simulink model "PowertaskEM22_Quadra"  (R2023b)
settings: Solver=VariableStepAuto  StartTime=0.0  StopTime=1  RelTol=1e-3
libraries: spsThreePhaseTransformerTwoWindingsLib x5, spsThreePhaseParallelRLCBranchLib x4, spsThreePhaseBreakerLib x4, spsThreePhaseVIMeasurementLib x4, spsRMSLib x4, spsThreePhaseSourceLib x3, sps_lib x1
settings Model: Creator=Shanilka T. Yapa  LastModifiedBy=Shanilka T. Yapa

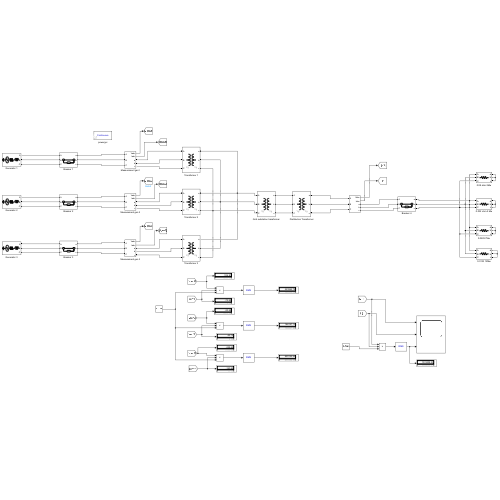
[thumbnail: Simulink's stored preview of the top-level diagram]
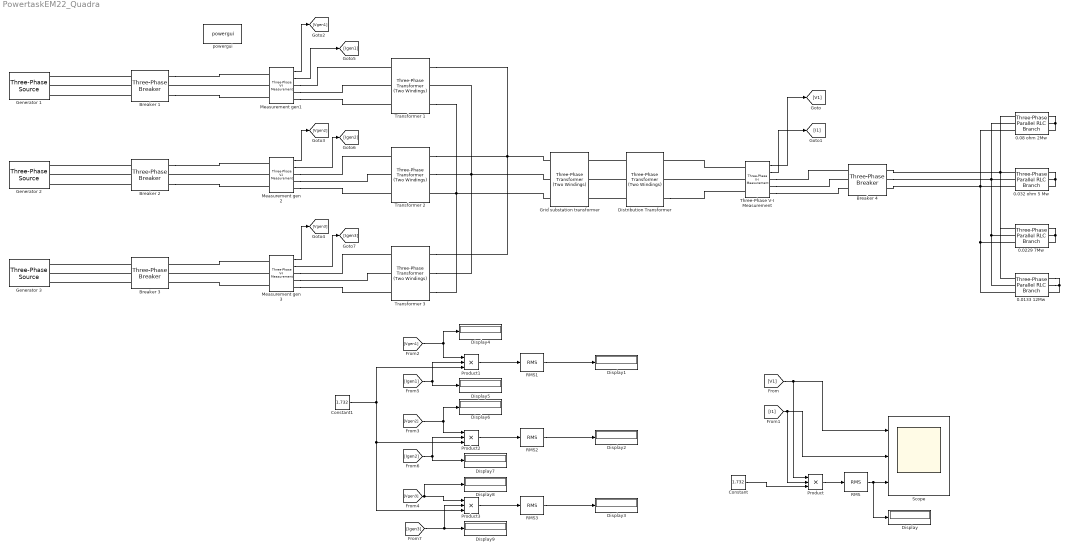
== system PowertaskEM22_Quadra ==
  0.0133 12Mw : spsThreePhaseParallelRLCBranchLib/Three-Phase Parallel RLC Branch  LConnTagsString=A|B|C  RConnTagsString=A|B|C  BranchType=R  Resistance=0.0133  Inductance=1e-3  Capacitance=1e-6  Measurements=None
  0.0229 7Mw : spsThreePhaseParallelRLCBranchLib/Three-Phase Parallel RLC Branch  LConnTagsString=A|B|C  RConnTagsString=A|B|C  BranchType=R  Resistance=0.0229  Inductance=1e-3  Capacitance=1e-6  Measurements=None
  0.032 ohm 5 Mw : spsThreePhaseParallelRLCBranchLib/Three-Phase Parallel RLC Branch  LConnTagsString=A|B|C  RConnTagsString=A|B|C  BranchType=R  Resistance=0.032  Inductance=0  Capacitance=0  Measurements=None
  0.08 ohm 2Mw : spsThreePhaseParallelRLCBranchLib/Three-Phase Parallel RLC Branch  LConnTagsString=A|B|C  RConnTagsString=A|B|C  BranchType=R  Resistance=0.08  Inductance=0  Capacitance=0  Measurements=None
  Breaker {1..4} (4 alike) : spsThreePhaseBreakerLib/Three-Phase Breaker  InitialState=closed  SwitchA=on  SwitchB=on  SwitchC=on  SwitchTimes="[1/60  5/60]"  External=off  BreakerResistance=0.01  SnubberResistance=1e6  SnubberCapacitance=inf  Measurements=None
  Constant : Constant  Value=1.732
  Constant1 : Constant  Value=1.732
  Display{,1..9} (10 alike) : Display
      settings: Format=bank
  Distribution Transformer : spsThreePhaseTransformerTwoWindingsLib/Three-Phase Transformer (Two Windings)  Winding1Connection=Yg  Winding2Connection=Yg  CoreType=Three single-phase transformers  SetSaturation=off  Hysteresis=off  DataFile='hysteresis'  SetInitialFlux=off  Measurements=None  UNITS=SI  NominalPower=[ 3e6 , 50 ]  Winding1=[11e3, 0.2, 0.006]  Winding2=[400, 0.001, 1e-4]  Rm=1e5  Lm=1e5  L0=0.5  Saturation=[0 0;0.66653 1910.3;277.72 2419.7]  InitialFluxes=[ 0.8 , -0.8 , 0.7 ]  BreakLoop=off  DiscreteSolver=Trapezoidal iterative  DataType=on  TransfoNumber=1
  Generator 1 : spsThreePhaseSourceLib/Three-Phase Source  InternalConnection=Yg  VoltagePhases=off  Voltage=11e3  PhaseAngle=0  Voltage_phases=[25e3 25e3 25e3]/sqrt(3)  PhaseAngles_phases=[0 -120 +120]  Frequency=50  NonIdealSource=on  SpecifyImpedance=off  Resistance=0.8929  Inductance=16.58e-3  ShortCircuitLevel=100e6  BaseVoltage=25e3  XRratio=7  BusType=PV  Pref=1e6  Qref=0  Prefabc=[10e3, 10e3, 10e3]  Qrefabc=[0, 0, 0]  Qmin=-inf  Qmax=inf
  Generator 2 : spsThreePhaseSourceLib/Three-Phase Source  InternalConnection=Yg  VoltagePhases=off  Voltage=12e3  PhaseAngle=0  Voltage_phases=[25e3 25e3 25e3]/sqrt(3)  PhaseAngles_phases=[0 -120 +120]  Frequency=50  NonIdealSource=on  SpecifyImpedance=off  Resistance=0.8929  Inductance=16.58e-3  ShortCircuitLevel=100e6  BaseVoltage=25e3  XRratio=7  BusType=PV  Pref=2e6  Qref=0  Prefabc=[10e3, 10e3, 10e3]  Qrefabc=[0, 0, 0]  Qmin=-inf  Qmax=inf
  Generator 3 : spsThreePhaseSourceLib/Three-Phase Source  InternalConnection=Yg  VoltagePhases=off  Voltage=10e3  PhaseAngle=0  Voltage_phases=[25e3 25e3 25e3]/sqrt(3)  PhaseAngles_phases=[0 -120 +120]  Frequency=50  NonIdealSource=on  SpecifyImpedance=off  Resistance=0.8929  Inductance=16.58e-3  ShortCircuitLevel=100e6  BaseVoltage=25e3  XRratio=7  BusType=PV  Pref=4e6  Qref=0  Prefabc=[10e3, 10e3, 10e3]  Qrefabc=[0, 0, 0]  Qmin=-inf  Qmax=inf
  Grid substation transformer : spsThreePhaseTransformerTwoWindingsLib/Three-Phase Transformer (Two Windings)  Winding1Connection=Yg  Winding2Connection=Yg  CoreType=Three single-phase transformers  SetSaturation=off  Hysteresis=off  DataFile='hysteresis'  SetInitialFlux=off  Measurements=None  UNITS=SI  NominalPower=[ 7e6 , 50 ]  Winding1=[132e3, 2, 0.06]  Winding2=[11e3, 0.2, 0.006]  Rm=1e5  Lm=1e5  L0=0.5  Saturation=[0 0;0.66653 1910.3;277.72 2419.7]  InitialFluxes=[ 0.8 , -0.8 , 0.7 ]  BreakLoop=off  DiscreteSolver=Trapezoidal iterative  DataType=on  TransfoNumber=1
  Measurement gen 2 : spsThreePhaseVIMeasurementLib/Three-Phase V-I Measurement  VoltageMeasurement=phase-to-ground  SetLabelV=off  LabelV=Vabc  Vpu=off  VpuLL=off  CurrentMeasurement=yes  SetLabelI=off  LabelI=Iabc  Ipu=off  Pbase=100e6  Vbase=500e3  OutputType=Complex  PhasorSimulation=off  PSBequivalent=0
  Measurement gen 3 : spsThreePhaseVIMeasurementLib/Three-Phase V-I Measurement  VoltageMeasurement=phase-to-ground  SetLabelV=off  LabelV=Vabc  Vpu=off  VpuLL=off  CurrentMeasurement=yes  SetLabelI=off  LabelI=Iabc  Ipu=off  Pbase=100e6  Vbase=500e3  OutputType=Complex  PhasorSimulation=off  PSBequivalent=0
  Measurement gen1 : spsThreePhaseVIMeasurementLib/Three-Phase V-I Measurement  VoltageMeasurement=phase-to-ground  SetLabelV=off  LabelV=Vabc  Vpu=off  VpuLL=off  CurrentMeasurement=yes  SetLabelI=off  LabelI=Iabc  Ipu=off  Pbase=100e6  Vbase=500e3  OutputType=Complex  PhasorSimulation=off  PSBequivalent=0
  Product{,1..3} (4 alike) : Product  Inputs=3
  RMS{,1..3} (4 alike) : spsRMSLib/RMS  TrueRMS=on  Freq=60  RMSInit=120  Ts=0
  Scope : Scope  NumInputPorts=3
  Three-Phase V-I Measurement : spsThreePhaseVIMeasurementLib/Three-Phase V-I Measurement  VoltageMeasurement=phase-to-phase  SetLabelV=off  LabelV=Vabc  Vpu=off  VpuLL=off  CurrentMeasurement=yes  SetLabelI=off  LabelI=Iabc  Ipu=off  Pbase=100e6  Vbase=500e3  OutputType=Complex  PhasorSimulation=off  PSBequivalent=0
  Transformer 1 : spsThreePhaseTransformerTwoWindingsLib/Three-Phase Transformer (Two Windings)  Winding1Connection=Yg  Winding2Connection=Yg  CoreType=Three single-phase transformers  SetSaturation=off  Hysteresis=off  DataFile='hysteresis'  SetInitialFlux=off  Measurements=None  UNITS=SI  NominalPower=[ 1e6 , 50 ]  Winding1=[11e3, 1.21, 0.04]  Winding2=[132e3, 16, 0.5]  Rm=1e5  Lm=1e5  L0=0.5  Saturation=[0 0;0.66653 1910.3;277.72 2419.7]  InitialFluxes=[ 0.8 , -0.8 , 0.7 ]  BreakLoop=off  DiscreteSolver=Trapezoidal iterative  DataType=on  TransfoNumber=1
  Transformer 2 : spsThreePhaseTransformerTwoWindingsLib/Three-Phase Transformer (Two Windings)  Winding1Connection=Yg  Winding2Connection=Yg  CoreType=Three single-phase transformers  SetSaturation=off  Hysteresis=off  DataFile='hysteresis'  SetInitialFlux=off  Measurements=None  UNITS=SI  NominalPower=[ 2e6 , 50 ]  Winding1=[12e3, 0.7, 0.2]  Winding2=[132e3, 8, 0.25]  Rm=1e5  Lm=1e5  L0=0.5  Saturation=[0 0;0.66653 1910.3;277.72 2419.7]  InitialFluxes=[ 0.8 , -0.8 , 0.7 ]  BreakLoop=off  DiscreteSolver=Trapezoidal iterative  DataType=on  TransfoNumber=1
  Transformer 3 : spsThreePhaseTransformerTwoWindingsLib/Three-Phase Transformer (Two Windings)  Winding1Connection=Yg  Winding2Connection=Yg  CoreType=Three single-phase transformers  SetSaturation=off  Hysteresis=off  DataFile='hysteresis'  SetInitialFlux=off  Measurements=None  UNITS=SI  NominalPower=[ 4e6 , 50 ]  Winding1=[10e3, 0.25,0.01]  Winding2=[132e3, 4, 0.125]  Rm=1e5  Lm=1e5  L0=0.5  Saturation=[0 0;0.66653 1910.3;277.72 2419.7]  InitialFluxes=[ 0.8 , -0.8 , 0.7 ]  BreakLoop=off  DiscreteSolver=Trapezoidal iterative  DataType=on  TransfoNumber=1
  powergui : sps_lib/powergui  Priority=1  SimulationMode=Continuous  SampleTime=50e-6  frequency=60  Iterations=50  frequencyindice=50  Pbase=100e6  ErrMax=1e-4  UnitsV=kV  UnitsW=MW  buscounter=0  FunctionMessages=off  echomessages=off  EnableUseOfTLC=off  CurrentSourceSwitches=off  DisableSnubberDevices=off  DisableRonSwitches=off  DisableVfSwitches=off  DisplayEquations=off  AutomaticDiscreteSolvers=off  SolverType=Tustin/Backward Euler (TBE)  Interpol=off  ExternalGateDelay=off  methode=off  Ts=100  x0status=blocks  SPID=on  SwTol=0  HookPort=off  NonlinearTolerance=1e-4  nMaxIteration=100  ContinueOnMaxIteration=off  RestoreLinks=warning  ResistiveCurrentMeasurement=off  Frange=[0:2:500]  Ylog=off  Xlog=on  ShowGrid=off  save=off  variable=ZData  structure=0  ZoomFFT=off  StartTime=0.0  cycles=1  DisplayStyle=1  fundamental=60  FreqAxis=off  MaxFrequency=1000  frequencyindicesteady=1  RmsSteady=1  display=off
  wires:
  Three-Phase V-I Measurement/1 -> [V1]
  Three-Phase V-I Measurement/2 -> [I1]
  [V1] -> Product/1, Scope/1
  [I1] -> Product/2, Scope/2
  Constant/1 -> Product/3
  Product/1 -> RMS/1
  RMS/1 -> Display/1, Scope/3
  Measurement gen1/1 -> [Vgen1]
  Measurement gen 2/1 -> [Vgen2]
  Measurement gen 3/1 -> [Vgen3]
  Measurement gen1/2 -> [Igen1]
  Measurement gen 2/2 -> [Igen2]
  Measurement gen 3/2 -> [Igen3]
  [Vgen1] -> Product1/1, Display4/1
  [Igen1] -> Product1/2, Display5/1
  Constant1/1 -> Product1/3, Product3/3, Product2/3
  [Vgen2] -> Product2/1, Display6/1
  [Igen2] -> Product2/2, Display7/1
  [Igen3] -> Display9/1, Product3/2
  Product3/1 -> RMS3/1
  Product2/1 -> RMS2/1
  Product1/1 -> RMS1/1
  RMS1/1 -> Display1/1
  RMS3/1 -> Display3/1
  RMS2/1 -> Display2/1
  [Vgen3] -> Display8/1, Product3/1
  connections:
  Transformer 1/RConn1 -- Transformer 3/RConn1 -- Grid substation transformer/LConn1 -- Transformer 2/RConn1
  Transformer 2/RConn2 -- Transformer 3/RConn2 -- Grid substation transformer/LConn2 -- Transformer 1/RConn2
  Transformer 1/RConn3 -- Transformer 3/RConn3 -- Grid substation transformer/LConn3 -- Transformer 2/RConn3
  Distribution Transformer/LConn1 -- Grid substation transformer/RConn1
  Distribution Transformer/LConn2 -- Grid substation transformer/RConn2
  Distribution Transformer/LConn3 -- Grid substation transformer/RConn3
  0.08 ohm 2Mw/LConn1 -- 0.0133 12Mw/LConn1 -- 0.0229 7Mw/LConn1 -- Breaker 4/RConn1 -- 0.032 ohm 5 Mw/LConn1
  0.08 ohm 2Mw/LConn2 -- Breaker 4/RConn2 -- 0.032 ohm 5 Mw/LConn2 -- 0.0133 12Mw/LConn2 -- 0.0229 7Mw/LConn2
  0.08 ohm 2Mw/LConn3 -- Breaker 4/RConn3 -- 0.032 ohm 5 Mw/LConn3 -- 0.0133 12Mw/LConn3 -- 0.0229 7Mw/LConn3
  Breaker 1/LConn1 -- Generator 1/RConn1
  Breaker 1/LConn2 -- Generator 1/RConn2
  Breaker 1/LConn3 -- Generator 1/RConn3
  Breaker 2/LConn1 -- Generator 2/RConn1
  Breaker 2/LConn2 -- Generator 2/RConn2
  Breaker 2/LConn3 -- Generator 2/RConn3
  Breaker 3/LConn2 -- Generator 3/RConn2
  Breaker 3/LConn1 -- Generator 3/RConn1
  Breaker 3/LConn3 -- Generator 3/RConn3
  Three-Phase V-I Measurement/LConn2 -- Distribution Transformer/RConn2
  Three-Phase V-I Measurement/LConn1 -- Distribution Transformer/RConn1
  Distribution Transformer/RConn3 -- Three-Phase V-I Measurement/LConn3
  Three-Phase V-I Measurement/RConn1 -- Breaker 4/LConn1
  Three-Phase V-I Measurement/RConn2 -- Breaker 4/LConn2
  Three-Phase V-I Measurement/RConn3 -- Breaker 4/LConn3
  0.08 ohm 2Mw/RConn1 -- 0.08 ohm 2Mw/RConn2 -- 0.08 ohm 2Mw/RConn3
  0.032 ohm 5 Mw/RConn1 -- 0.032 ohm 5 Mw/RConn2 -- 0.032 ohm 5 Mw/RConn3
  0.0229 7Mw/RConn1 -- 0.0229 7Mw/RConn2 -- 0.0229 7Mw/RConn3
  0.0133 12Mw/RConn1 -- 0.0133 12Mw/RConn2 -- 0.0133 12Mw/RConn3
  Measurement gen1/LConn2 -- Breaker 1/RConn2
  Measurement gen1/RConn2 -- Transformer 1/LConn2
  Measurement gen1/RConn1 -- Transformer 1/LConn1
  Measurement gen1/RConn3 -- Transformer 1/LConn3
  Breaker 1/RConn1 -- Measurement gen1/LConn1
  Breaker 1/RConn3 -- Measurement gen1/LConn3
  Measurement gen 2/LConn2 -- Breaker 2/RConn2
  Breaker 2/RConn1 -- Measurement gen 2/LConn1
  Breaker 2/RConn3 -- Measurement gen 2/LConn3
  Measurement gen 2/RConn1 -- Transformer 2/LConn1
  Measurement gen 2/RConn2 -- Transformer 2/LConn2
  Measurement gen 2/RConn3 -- Transformer 2/LConn3
  Measurement gen 3/LConn2 -- Breaker 3/RConn2
  Measurement gen 3/RConn1 -- Transformer 3/LConn1
  Measurement gen 3/RConn2 -- Transformer 3/LConn2
  Measurement gen 3/RConn3 -- Transformer 3/LConn3
  Measurement gen 3/LConn1 -- Breaker 3/RConn1
  Measurement gen 3/LConn3 -- Breaker 3/RConn3
